simulink library "halout"  (R2021b)
settings: Solver=VariableStepAuto  StartTime=0.0  StopTime=10.0  RelTol=1e-3
undefined symbols (not defined in the file): C_TASK_5MS_S, FALSE, KHAL_CAN1FDAPS3E2E_flg, KHAL_CAN1FDAPS3TxReq_flg, KHAL_CAN1FDVCU2E2E_flg, KHAL_CAN1FDVCU2TxReq_flg, KHAL_CAN1FDVCU3E2E_flg, KHAL_CAN1FDVCU3TxReq_flg, KHAL_CAN1TxReq_flg, KHAL_CAN2TxReq_flg, KHAL_CAN3FDVCU1TxReq_flg, KHAL_CAN3FDVCU2E2E_flg, KHAL_CAN3FDVCU2TxReq_flg, KHAL_CAN3TxReq_flg, KHAL_CAN4FDVCU1E2E_flg, KHAL_CAN4FDVCU1TxReq_flg, KHAL_CAN4TxReq_flg, KHAL_CAN5TxReq_flg, ONE_INT, TRUE, ZERO_INT
libraries: FVT_lib x383, simulink x179
(part 11 of 20)

== system halout/HAL_OUT/CAN5/FD_VCU0_0x1F0 ==
  BSCP_outputs : Inport  OutDataTypeStr=Bus: BSCP_outputs
  BOUTP_outputs : Inport  Port=2  OutDataTypeStr=Bus: BOUTP_outputs
  EVCCAplusPwrUpReq : Subsystem
  FDADC12VDetAvg : Subsystem
  FrTqSource : Subsystem
  Ground{,1..8} (9 alike) : Ground
  HVRlyOpFail : Subsystem
  HVTHCMSysAvail : Subsystem
  LVBattChrgtimeAct : Subsystem
  LVBattVoltSta : Subsystem
  LVChrgHoldTAct : Subsystem
  LVSilentChrgLv : Subsystem
  LVSilentChrgReq : Subsystem
  LVSilentChrgSta : Subsystem
  MCUActDisFail : Subsystem
  PMMAllowECUSleep : Subsystem
  PowerDownFault : Subsystem
  PowerDownState : Subsystem
  PowerUpFault : Subsystem
  PowerUpState : Subsystem
  PwrDownReq : Subsystem
  PwrStaConstraint : Subsystem
  PwrStaONTOIVIPopReq : Subsystem
  PwrStaONTOIVIPopT : Subsystem
  PwrStaSelect : Subsystem
  PwrStaTOSta : Subsystem
  PwrUpReq : Subsystem
  RrTqSource : Subsystem
  SchedChgTOSta : Subsystem
  SilentChkAllowSleep : Subsystem
  SysAllowReadySta : Subsystem
  SysPwrSta : Subsystem
  TCountSta : Subsystem
  TimerAllowSleep : Subsystem
  VCUBrkSWSta : Subsystem
  VCUFLDoorSta : Subsystem
  VCUFRDoorSta : Subsystem
  VCURLDoorSta : Subsystem
  VCURRDoorSta : Subsystem
  VehHVPwrAvail4THCM : Subsystem
  bus_creator : BusCreator  Inputs=37  OutDataTypeStr=Bus: DT_CAN5_SG_FD_VCU0  NonVirtualBus=on
  bus_selector : BusSelector  OutputSignals=VOUTP_EvccAplusPwrUpReq_flg
  bus_selector1 : BusSelector  OutputSignals=VOUTP_FDADC12VDetAvg_mV
  bus_selector10 : BusSelector  OutputSignals=VOUTP_PMMAllowECUSleep_flg
  bus_selector11 : BusSelector  OutputSignals=VOUTP_PowerDownFault_enum
  bus_selector12 : BusSelector  OutputSignals=VOUTP_PowerDownState_enum
  bus_selector13 : BusSelector  OutputSignals=VOUTP_PowerUpFault_enum
  bus_selector14 : BusSelector  OutputSignals=VOUTP_PowerUpState_enum
  bus_selector15 : BusSelector  OutputSignals=VOUTP_PwrDownReq_enum
  bus_selector16 : BusSelector  OutputSignals=VOUTP_PwrStaConstraint_enum
  bus_selector17 : BusSelector  OutputSignals=VOUTP_PwrStaONTOPopReq_flg
  bus_selector18 : BusSelector  OutputSignals=VOUTP_IVIPwrStaONTOPopT_s
  bus_selector19 : BusSelector  OutputSignals=VOUTP_PwrStaSelect_enum
  bus_selector2 : BusSelector  OutputSignals=VOUTP_TqSourceFr_enum
  bus_selector20 : BusSelector  OutputSignals=VOUTP_PwrStaTOSta_enum
  bus_selector21 : BusSelector  OutputSignals=VOUTP_PwrUpReq_enum
  bus_selector22 : BusSelector  OutputSignals=VOUTP_TqSourceRr_enum
  bus_selector23 : BusSelector  OutputSignals=VOUTP_SilentChkAllowSleep_flg
  bus_selector24 : BusSelector  OutputSignals=VOUTP_SysPowerMode_enum
  bus_selector25 : BusSelector  OutputSignals=VOUTP_TCountSta_enum
  bus_selector26 : BusSelector  OutputSignals=VOUTP_TimerAllowSleep_flg
  bus_selector27 : BusSelector  OutputSignals=VOUTP_VehHVPwrAvail4THCM_W
  bus_selector3 : BusSelector  OutputSignals=VOUTP_HVTHCMSysAvail_enum
  bus_selector4 : BusSelector  OutputSignals=VOUTP_LVBattChrgTimeCnt_s
  bus_selector5 : BusSelector  OutputSignals=VOUTP_LVBattVoltSta_enum
  bus_selector6 : BusSelector  OutputSignals=VOUTP_LVChrgHoldTtimer_s
  bus_selector7 : BusSelector  OutputSignals=VOUTP_LVSilentChrgLv_enum
  bus_selector8 : BusSelector  OutputSignals=VOUTP_LVSilentChrgReq_flg
  bus_selector9 : BusSelector  OutputSignals=VOUTP_LVSilentChrgSta_enum
  FD_VCU0 : Outport
  wires:
  BSCP_outputs/1 -> [BSCP_outputs]
  BOUTP_outputs/1 -> [BOUTP_outputs]
  [CAN5_EVCCAplusPwrUpReq] -> bus_creator/1  "CAN5_EVCCAplusPwrUpReq"
  [CAN5_FDADC12VDetAvg] -> bus_creator/2  "CAN5_FDADC12VDetAvg"
  [CAN5_Fr_TqSource] -> bus_creator/3  "CAN5_Fr_TqSource"
  [CAN5_HVRlyOpFail] -> bus_creator/4  "CAN5_HVRlyOpFail"
  [CAN5_HVTHCMSysAvail] -> bus_creator/5  "CAN5_HVTHCMSysAvail"
  [CAN5_LVBattChrgtimeAct] -> bus_creator/6  "CAN5_LVBattChrgtimeAct"
  [CAN5_LVBattVoltSta] -> bus_creator/7  "CAN5_LVBattVoltSta"
  [CAN5_LVChrgHoldTAct] -> bus_creator/8  "CAN5_LVChrgHoldTAct"
  [CAN5_LVSilentChrgLv] -> bus_creator/9  "CAN5_LVSilentChrgLv"
  [CAN5_LVSilentChrgReq] -> bus_creator/10  "CAN5_LVSilentChrgReq"
  [CAN5_LVSilentChrgSta] -> bus_creator/11  "CAN5_LVSilentChrgSta"
  [CAN5_MCUActDisFail] -> bus_creator/12  "CAN5_MCUActDisFail"
  [CAN5_PMMAllowECUSleep] -> bus_creator/13  "CAN5_PMMAllowECUSleep"
  [CAN5_PowerDownFault] -> bus_creator/14  "CAN5_PowerDownFault"
  [CAN5_PowerDownState] -> bus_creator/15  "CAN5_PowerDownState"
  [CAN5_PowerUpFault] -> bus_creator/16  "CAN5_PowerUpFault"
  [CAN5_PowerUpState] -> bus_creator/17  "CAN5_PowerUpState"
  [CAN5_PwrDownReq] -> bus_creator/18  "CAN5_PwrDownReq"
  [CAN5_PwrStaConstraint] -> bus_creator/19  "CAN5_PwrStaConstraint"
  [CAN5_PwrStaONTOIVIPopReq] -> bus_creator/20  "CAN5_PwrStaONTOIVIPopReq"
  [CAN5_PwrStaONTOIVIPopT] -> bus_creator/21  "CAN5_PwrStaONTOIVIPopT"
  [CAN5_PwrStaSelect] -> bus_creator/22  "CAN5_PwrStaSelect"
  [CAN5_PwrStaTOSta] -> bus_creator/23  "CAN5_PwrStaTOSta"
  [CAN5_PwrUpReq] -> bus_creator/24  "CAN5_PwrUpReq"
  [CAN5_Rr_TqSource] -> bus_creator/25  "CAN5_Rr_TqSource"
  [CAN5_SchedChgTOSta] -> bus_creator/26  "CAN5_SchedChgTOSta"
  [CAN5_SilentChkAllowSleep] -> bus_creator/27  "CAN5_SilentChkAllowSleep"
  [CAN5_SysAllowReadySta] -> bus_creator/28  "CAN5_SysAllowReadySta"
  [CAN5_SysPwrSta] -> bus_creator/29  "CAN5_SysPwrSta"
  [CAN5_TCountSta] -> bus_creator/30  "CAN5_TCountSta"
  [CAN5_TimerAllowSleep] -> bus_creator/31  "CAN5_TimerAllowSleep"
  [CAN5_VCUBrkSWSta] -> bus_creator/32  "CAN5_VCUBrkSWSta"
  [CAN5_VCUFLDoorSta] -> bus_creator/33  "CAN5_VCUFLDoorSta"
  [CAN5_VCUFRDoorSta] -> bus_creator/34  "CAN5_VCUFRDoorSta"
  [CAN5_VCURLDoorSta] -> bus_creator/35  "CAN5_VCURLDoorSta"
  [CAN5_VCURRDoorSta] -> bus_creator/36  "CAN5_VCURRDoorSta"
  [CAN5_VehHVPwrAvail4THCM] -> bus_creator/37  "CAN5_VehHVPwrAvail4THCM"
  bus_creator/1 -> FD_VCU0/1
  EVCCAplusPwrUpReq/1(CAN5_EVCCAplusPwrUpReq) -> [CAN5_EVCCAplusPwrUpReq]
  FDADC12VDetAvg/1(CAN5_FDADC12VDetAvg) -> [CAN5_FDADC12VDetAvg]
  FrTqSource/1(CAN5_Fr_TqSource) -> [CAN5_Fr_TqSource]
  HVRlyOpFail/1(CAN5_HVRlyOpFail) -> [CAN5_HVRlyOpFail]
  HVTHCMSysAvail/1(CAN5_HVTHCMSysAvail) -> [CAN5_HVTHCMSysAvail]
  LVBattChrgtimeAct/1(CAN5_LVBattChrgtimeAct) -> [CAN5_LVBattChrgtimeAct]
  LVBattVoltSta/1(CAN5_LVBattVoltSta) -> [CAN5_LVBattVoltSta]
  LVChrgHoldTAct/1(CAN5_LVChrgHoldTAct) -> [CAN5_LVChrgHoldTAct]
  LVSilentChrgLv/1(CAN5_LVSilentChrgLv) -> [CAN5_LVSilentChrgLv]
  LVSilentChrgReq/1(CAN5_LVSilentChrgReq) -> [CAN5_LVSilentChrgReq]
  LVSilentChrgSta/1(CAN5_LVSilentChrgSta) -> [CAN5_LVSilentChrgSta]
  MCUActDisFail/1(CAN5_MCUActDisFail) -> [CAN5_MCUActDisFail]
  PMMAllowECUSleep/1(CAN5_PMMAllowECUSleep) -> [CAN5_PMMAllowECUSleep]
  PowerDownFault/1(CAN5_PowerDownFault) -> [CAN5_PowerDownFault]
  PowerDownState/1(CAN5_PowerDownState) -> [CAN5_PowerDownState]
  PowerUpFault/1(CAN5_PowerUpFault) -> [CAN5_PowerUpFault]
  PowerUpState/1(CAN5_PowerUpState) -> [CAN5_PowerUpState]
  PwrDownReq/1(CAN5_PwrDownReq) -> [CAN5_PwrDownReq]
  PwrStaConstraint/1(CAN5_PwrStaConstraint) -> [CAN5_PwrStaConstraint]
  PwrStaONTOIVIPopReq/1(CAN5_PwrStaONTOIVIPopReq) -> [CAN5_PwrStaONTOIVIPopReq]
  PwrStaONTOIVIPopT/1(CAN5_PwrStaONTOIVIPopT) -> [CAN5_PwrStaONTOIVIPopT]
  PwrStaSelect/1(CAN5_PwrStaSelect) -> [CAN5_PwrStaSelect]
  PwrStaTOSta/1(CAN5_PwrStaTOSta) -> [CAN5_PwrStaTOSta]
  PwrUpReq/1(CAN5_PwrUpReq) -> [CAN5_PwrUpReq]
  RrTqSource/1(CAN5_Rr_TqSource) -> [CAN5_Rr_TqSource]
  SchedChgTOSta/1(CAN5_SchedChgTOSta) -> [CAN5_SchedChgTOSta]
  SilentChkAllowSleep/1(CAN5_SilentChkAllowSleep) -> [CAN5_SilentChkAllowSleep]
  SysAllowReadySta/1(CAN5_SysAllowReadySta) -> [CAN5_SysAllowReadySta]
  SysPwrSta/1(CAN5_SysPwrSta) -> [CAN5_SysPwrSta]
  TCountSta/1(CAN5_TCountSta) -> [CAN5_TCountSta]
  TimerAllowSleep/1(CAN5_TimerAllowSleep) -> [CAN5_TimerAllowSleep]
  VCUBrkSWSta/1(CAN5_VCUBrkSWSta) -> [CAN5_VCUBrkSWSta]
  VCUFLDoorSta/1(CAN5_VCUFLDoorSta) -> [CAN5_VCUFLDoorSta]
  VCUFRDoorSta/1(CAN5_VCUFRDoorSta) -> [CAN5_VCUFRDoorSta]
  VCURLDoorSta/1(CAN5_VCURLDoorSta) -> [CAN5_VCURLDoorSta]
  VCURRDoorSta/1(CAN5_VCURRDoorSta) -> [CAN5_VCURRDoorSta]
  VehHVPwrAvail4THCM/1(CAN5_VehHVPwrAvail4THCM) -> [CAN5_VehHVPwrAvail4THCM]
  bus_selector/1 -> EVCCAplusPwrUpReq/1(EVCCAplusPwrUpReq)  "<VOUTP_EvccAplusPwrUpReq_flg>"
  [BOUTP_outputs] -> bus_selector/1
  bus_selector1/1 -> FDADC12VDetAvg/1(FDADC12VDetAvg)  "<VOUTP_FDADC12VDetAvg_mV>"
  [BOUTP_outputs] -> bus_selector1/1
  bus_selector2/1 -> FrTqSource/1(FrTqSource)  "<VOUTP_TqSourceFr_enum>"
  [BOUTP_outputs] -> bus_selector2/1
  Ground/1 -> HVRlyOpFail/1(HVRlyOpFail)
  bus_selector3/1 -> HVTHCMSysAvail/1(HVTHCMSysAvail)  "<VOUTP_HVTHCMSysAvail_enum>"
  [BOUTP_outputs] -> bus_selector3/1
  bus_selector4/1 -> LVBattChrgtimeAct/1(LVBattChrgtimeAct)  "<VOUTP_LVBattChrgTimeCnt_s>"
  [BOUTP_outputs] -> bus_selector4/1
  bus_selector5/1 -> LVBattVoltSta/1(LVBattVoltSta)  "<VOUTP_LVBattVoltSta_enum>"
  [BOUTP_outputs] -> bus_selector5/1
  bus_selector6/1 -> LVChrgHoldTAct/1(LVChrgHoldTAct)  "<VOUTP_LVChrgHoldTtimer_s>"
  [BOUTP_outputs] -> bus_selector6/1
  bus_selector7/1 -> LVSilentChrgLv/1(LVSilentChrgLv)  "<VOUTP_LVSilentChrgLv_enum>"
  [BOUTP_outputs] -> bus_selector7/1
  bus_selector8/1 -> LVSilentChrgReq/1(LVSilentChrgReq)  "<VOUTP_LVSilentChrgReq_flg>"
  [BOUTP_outputs] -> bus_selector8/1
  bus_selector9/1 -> LVSilentChrgSta/1(LVSilentChrgSta)  "<VOUTP_LVSilentChrgSta_enum>"
  [BOUTP_outputs] -> bus_selector9/1
  Ground1/1 -> MCUActDisFail/1(MCUActDisFail)
  bus_selector10/1 -> PMMAllowECUSleep/1(PMMAllowECUSleep)  "<VOUTP_PMMAllowECUSleep_flg>"
  [BOUTP_outputs] -> bus_selector10/1
  bus_selector11/1 -> PowerDownFault/1(PowerDownFault)  "<VOUTP_PowerDownFault_enum>"
  [BOUTP_outputs] -> bus_selector11/1
  bus_selector12/1 -> PowerDownState/1(PowerDownState)  "<VOUTP_PowerDownState_enum>"
  [BOUTP_outputs] -> bus_selector12/1
  bus_selector13/1 -> PowerUpFault/1(PowerUpFault)  "<VOUTP_PowerUpFault_enum>"
  [BOUTP_outputs] -> bus_selector13/1
  bus_selector14/1 -> PowerUpState/1(PowerUpState)  "<VOUTP_PowerUpState_enum>"
  [BOUTP_outputs] -> bus_selector14/1
  bus_selector15/1 -> PwrDownReq/1(PwrDownReq)  "<VOUTP_PwrDownReq_enum>"
  [BOUTP_outputs] -> bus_selector15/1
  bus_selector16/1 -> PwrStaConstraint/1(PwrStaConstraint)  "<VOUTP_PwrStaConstraint_enum>"
  [BOUTP_outputs] -> bus_selector16/1
  bus_selector17/1 -> PwrStaONTOIVIPopReq/1(PwrStaONTOIVIPopReq)  "<VOUTP_PwrStaONTOPopReq_flg>"
  [BOUTP_outputs] -> bus_selector17/1
  bus_selector18/1 -> PwrStaONTOIVIPopT/1(PwrStaONTOIVIPopT)  "<VOUTP_IVIPwrStaONTOPopT_s>"
  [BOUTP_outputs] -> bus_selector18/1
  bus_selector19/1 -> PwrStaSelect/1(PwrStaSelect)  "<VOUTP_PwrStaSelect_enum>"
  [BOUTP_outputs] -> bus_selector19/1
  bus_selector20/1 -> PwrStaTOSta/1(PwrStaTOSta)  "<VOUTP_PwrStaTOSta_enum>"
  [BOUTP_outputs] -> bus_selector20/1
  bus_selector21/1 -> PwrUpReq/1(PwrUpReq)  "<VOUTP_PwrUpReq_enum>"
  [BOUTP_outputs] -> bus_selector21/1
  bus_selector22/1 -> RrTqSource/1(RrTqSource)  "<VOUTP_TqSourceRr_enum>"
  [BOUTP_outputs] -> bus_selector22/1
  Ground2/1 -> SchedChgTOSta/1(SchedChgTOSta)
  bus_selector23/1 -> SilentChkAllowSleep/1(SilentChkAllowSleep)  "<VOUTP_SilentChkAllowSleep_flg>"
  [BOUTP_outputs] -> bus_selector23/1
  Ground3/1 -> SysAllowReadySta/1(SysAllowReadySta)
  bus_selector24/1 -> SysPwrSta/1(SysPwrSta)  "<VOUTP_SysPowerMode_enum>"
  [BOUTP_outputs] -> bus_selector24/1
  bus_selector25/1 -> TCountSta/1(TCountSta)  "<VOUTP_TCountSta_enum>"
  [BOUTP_outputs] -> bus_selector25/1
  bus_selector26/1 -> TimerAllowSleep/1(TimerAllowSleep)  "<VOUTP_TimerAllowSleep_flg>"
  [BOUTP_outputs] -> bus_selector26/1
  Ground4/1 -> VCUBrkSWSta/1(VCUBrkSWSta)
  Ground5/1 -> VCUFLDoorSta/1(VCUFLDoorSta)
  Ground6/1 -> VCUFRDoorSta/1(VCUFRDoorSta)
  Ground7/1 -> VCURLDoorSta/1(VCURLDoorSta)
  Ground8/1 -> VCURRDoorSta/1(VCURRDoorSta)
  bus_selector27/1 -> VehHVPwrAvail4THCM/1(VehHVPwrAvail4THCM)  "<VOUTP_VehHVPwrAvail4THCM_W>"
  [BOUTP_outputs] -> bus_selector27/1

== system halout/HAL_OUT/CAN5/FD_VCU1_0x116 ==
  BSCP_outputs : Inport  OutDataTypeStr=Bus: BSCP_outputs
  BOUTP_outputs : Inport  Port=2  OutDataTypeStr=Bus: BOUTP_outputs
  MSACrlSta : Subsystem
  PwrSta : Subsystem
  ShiftGearPosn : Subsystem
  bus_creator : BusCreator  Inputs=3  OutDataTypeStr=Bus: DT_CAN5_SG_FD_VCU1  NonVirtualBus=on
  bus_selector : BusSelector  OutputSignals=VOUTP_MSACtrlSta_enum
  bus_selector1 : BusSelector  OutputSignals=VOUTP_PowerSta_enum
  bus_selector2 : BusSelector  OutputSignals=VOUTP_ShiftGearPosn_enum
  FD_VCU1 : Outport
  wires:
  BSCP_outputs/1 -> [BSCP_outputs]
  BOUTP_outputs/1 -> [BOUTP_outputs]
  [CAN5_MSA_Crl_Sta] -> bus_creator/1  "CAN5_MSA_Crl_Sta"
  [CAN5_PwrSta] -> bus_creator/2  "CAN5_PwrSta"
  [CAN5_ShiftGearPosn] -> bus_creator/3  "CAN5_ShiftGearPosn"
  bus_creator/1 -> FD_VCU1/1
  MSACrlSta/1(CAN5_MSA_Crl_Sta) -> [CAN5_MSA_Crl_Sta]
  PwrSta/1(CAN5_PwrSta) -> [CAN5_PwrSta]
  ShiftGearPosn/1(CAN5_ShiftGearPosn) -> [CAN5_ShiftGearPosn]
  bus_selector/1 -> MSACrlSta/1(MSACrlSta)  "<VOUTP_MSACtrlSta_enum>"
  [BOUTP_outputs] -> bus_selector/1
  bus_selector1/1 -> PwrSta/1(PwrSta)  "<VOUTP_PowerSta_enum>"
  [BOUTP_outputs] -> bus_selector1/1
  bus_selector2/1 -> ShiftGearPosn/1(ShiftGearPosn)  "<VOUTP_ShiftGearPosn_enum>"
  [BOUTP_outputs] -> bus_selector2/1

== system halout/HAL_OUT/CAN5/FD_VCU3_0x159 ==
  BSCP_outputs : Inport  OutDataTypeStr=Bus: BSCP_outputs
  BOUTP_outputs : Inport  Port=2  OutDataTypeStr=Bus: BOUTP_outputs
  CSVCU3CAN1 : Subsystem
  EquivAccPedalSWSta : Subsystem
  FrEDUActTqValid : Subsystem
  FrEDUAvailBrkRgnTq : Subsystem
  FrEDUAvailBrkRgnTqValid : Subsystem
  FrEDURealARgnTq : Subsystem
  FrEDURealDrvOrBRgnTq : Subsystem
  FrEDURolRgnTqValid : Subsystem
  FrEDUSpd : Subsystem
  FrEDUSpdValid : Subsystem
  FrRgnDecrSta : Subsystem
  FrRgnPermSta : Subsystem
  Ground{,1..5} (6 alike) : Ground
  PTCSPermSta : Subsystem
  RCVCU3CAN1 : Subsystem
  RgnAbnorSta : Subsystem
  RrEDUActTqValid : Subsystem
  RrEDUAvailBrkRgnTq : Subsystem
  RrEDUAvailBrkRgnTqValid : Subsystem
  RrEDURealARgnTq : Subsystem
  RrEDURealDrvOrBRgnTq : Subsystem
  RrEDURolRgnTqValid : Subsystem
  RrEDUSpd : Subsystem
  RrEDUSpdValid : Subsystem
  RrRgnDecrSta : Subsystem
  RrRgnPermSta : Subsystem
  bus_creator : BusCreator  Inputs=25  OutDataTypeStr=Bus: DT_CAN5_SG_FD_VCU3  NonVirtualBus=on
  bus_selector : BusSelector  OutputSignals=VOUTP_EquivAccPedalSWSta_flg
  bus_selector1 : BusSelector  OutputSignals=VOUTP_FrEDUAvailBrkRgnTq_Nm
  bus_selector10 : BusSelector  OutputSignals=VOUTP_RgnAbnorSta_flg
  bus_selector11 : BusSelector  OutputSignals=VOUTP_RrEDUAvailBrkRgnTq_Nm
  bus_selector12 : BusSelector  OutputSignals=VOUTP_RrEDUAvailBrkRgnTqV_flg
  bus_selector13 : BusSelector  OutputSignals=VOUTP_RrEDURolRgnTq_Nm
  bus_selector14 : BusSelector  OutputSignals=VOUTP_RrEDUActTq_Nm
  bus_selector15 : BusSelector  OutputSignals=VOUTP_RrEDUSpd_rpm
  bus_selector16 : BusSelector  OutputSignals=VOUTP_RrEDUSpdValid_flg
  bus_selector17 : BusSelector  OutputSignals=VOUTP_RrRgnDecrSta_flg
  bus_selector18 : BusSelector  OutputSignals=VOUTP_RrRgnPermSta_flg
  bus_selector2 : BusSelector  OutputSignals=VOUTP_FrEDUAvailBrkRgnTqV_flg
  bus_selector3 : BusSelector  OutputSignals=VOUTP_FrEDURolRgnTq_Nm
  bus_selector4 : BusSelector  OutputSignals=VOUTP_FrEDUActTq_Nm
  bus_selector5 : BusSelector  OutputSignals=VOUTP_FrEDUSpd_rpm
  bus_selector6 : BusSelector  OutputSignals=VOUTP_FrEDUSpdValid_flg
  bus_selector7 : BusSelector  OutputSignals=VOUTP_FrRgnDecrSta_flg
  bus_selector8 : BusSelector  OutputSignals=VOUTP_FrRgnPermSta_flg
  bus_selector9 : BusSelector  OutputSignals=VOUTP_PTCSPermSta_flg
  FD_VCU3 : Outport
  wires:
  BSCP_outputs/1 -> [BSCP_outputs]
  BOUTP_outputs/1 -> [BOUTP_outputs]
  [CAN5_CS_VCU3_CAN1] -> bus_creator/1  "CAN5_CS_VCU3_CAN1"
  [CAN5_EquivAccPedalSWSta] -> bus_creator/2  "CAN5_EquivAccPedalSWSta"
  [CAN5_Fr_EDUActTqValid] -> bus_creator/3  "CAN5_Fr_EDUActTqValid"
  [CAN5_Fr_EDUAvailBrkRgnTq] -> bus_creator/4  "CAN5_Fr_EDUAvailBrkRgnTq"
  [CAN5_Fr_EDUAvailBrkRgnTqValid] -> bus_creator/5  "CAN5_Fr_EDUAvailBrkRgnTqValid"
  [CAN5_Fr_EDURealARgnTq] -> bus_creator/6  "CAN5_Fr_EDURealARgnTq"
  [CAN5_Fr_EDURealDrvOrBRgnTq] -> bus_creator/7  "CAN5_Fr_EDURealDrvOrBRgnTq"
  [CAN5_Fr_EDURolRgnTqValid] -> bus_creator/8  "CAN5_Fr_EDURolRgnTqValid"
  [CAN5_Fr_EDUSpd] -> bus_creator/9  "CAN5_Fr_EDUSpd"
  [CAN5_Fr_EDUSpdValid] -> bus_creator/10  "CAN5_Fr_EDUSpdValid"
  [CAN5_Fr_RgnDecrSta] -> bus_creator/11  "CAN5_Fr_RgnDecrSta"
  [CAN5_Fr_RgnPermSta] -> bus_creator/12  "CAN5_Fr_RgnPermSta"
  [CAN5_PTCS_PermSta] -> bus_creator/13  "CAN5_PTCS_PermSta"
  [CAN5_RC_VCU3_CAN1] -> bus_creator/14  "CAN5_RC_VCU3_CAN1"
  [CAN5_RgnAbnorSta] -> bus_creator/15  "CAN5_RgnAbnorSta"
  [CAN5_Rr_EDUActTqValid] -> bus_creator/16  "CAN5_Rr_EDUActTqValid"
  [CAN5_Rr_EDUAvailBrkRgnTq] -> bus_creator/17  "CAN5_Rr_EDUAvailBrkRgnTq"
  [CAN5_Rr_EDUAvailBrkRgnTqValid] -> bus_creator/18  "CAN5_Rr_EDUAvailBrkRgnTqValid"
  [CAN5_Rr_EDURealARgnTq] -> bus_creator/19  "CAN5_Rr_EDURealARgnTq"
  [CAN5_Rr_EDURealDrvOrBRgnTq] -> bus_creator/20  "CAN5_Rr_EDURealDrvOrBRgnTq"
  [CAN5_Rr_EDURolRgnTqValid] -> bus_creator/21  "CAN5_Rr_EDURolRgnTqValid"
  [CAN5_Rr_EDUSpd] -> bus_creator/22  "CAN5_Rr_EDUSpd"
  [CAN5_Rr_EDUSpdValid] -> bus_creator/23  "CAN5_Rr_EDUSpdValid"
  [CAN5_Rr_RgnDecrSta] -> bus_creator/24  "CAN5_Rr_RgnDecrSta"
  [CAN5_Rr_RgnPermSta] -> bus_creator/25  "CAN5_Rr_RgnPermSta"
  bus_creator/1 -> FD_VCU3/1
  CSVCU3CAN1/1(CAN5_CS_VCU3_CAN1) -> [CAN5_CS_VCU3_CAN1]
  EquivAccPedalSWSta/1(CAN5_EquivAccPedalSWSta) -> [CAN5_EquivAccPedalSWSta]
  FrEDUActTqValid/1(CAN5_Fr_EDUActTqValid) -> [CAN5_Fr_EDUActTqValid]
  FrEDUAvailBrkRgnTq/1(CAN5_Fr_EDUAvailBrkRgnTq) -> [CAN5_Fr_EDUAvailBrkRgnTq]
  FrEDUAvailBrkRgnTqValid/1(CAN5_Fr_EDUAvailBrkRgnTqValid) -> [CAN5_Fr_EDUAvailBrkRgnTqValid]
  FrEDURealARgnTq/1(CAN5_Fr_EDURealARgnTq) -> [CAN5_Fr_EDURealARgnTq]
  FrEDURealDrvOrBRgnTq/1(CAN5_Fr_EDURealDrvOrBRgnTq) -> [CAN5_Fr_EDURealDrvOrBRgnTq]
  FrEDURolRgnTqValid/1(CAN5_Fr_EDURolRgnTqValid) -> [CAN5_Fr_EDURolRgnTqValid]
  FrEDUSpd/1(CAN5_Fr_EDUSpd) -> [CAN5_Fr_EDUSpd]
  FrEDUSpdValid/1(CAN5_Fr_EDUSpdValid) -> [CAN5_Fr_EDUSpdValid]
  FrRgnDecrSta/1(CAN5_Fr_RgnDecrSta) -> [CAN5_Fr_RgnDecrSta]
  FrRgnPermSta/1(CAN5_Fr_RgnPermSta) -> [CAN5_Fr_RgnPermSta]
  PTCSPermSta/1(CAN5_PTCS_PermSta) -> [CAN5_PTCS_PermSta]
  RCVCU3CAN1/1(CAN5_RC_VCU3_CAN1) -> [CAN5_RC_VCU3_CAN1]
  RgnAbnorSta/1(CAN5_RgnAbnorSta) -> [CAN5_RgnAbnorSta]
  RrEDUActTqValid/1(CAN5_Rr_EDUActTqValid) -> [CAN5_Rr_EDUActTqValid]
  RrEDUAvailBrkRgnTq/1(CAN5_Rr_EDUAvailBrkRgnTq) -> [CAN5_Rr_EDUAvailBrkRgnTq]
  RrEDUAvailBrkRgnTqValid/1(CAN5_Rr_EDUAvailBrkRgnTqValid) -> [CAN5_Rr_EDUAvailBrkRgnTqValid]
  RrEDURealARgnTq/1(CAN5_Rr_EDURealARgnTq) -> [CAN5_Rr_EDURealARgnTq]
  RrEDURealDrvOrBRgnTq/1(CAN5_Rr_EDURealDrvOrBRgnTq) -> [CAN5_Rr_EDURealDrvOrBRgnTq]
  RrEDURolRgnTqValid/1(CAN5_Rr_EDURolRgnTqValid) -> [CAN5_Rr_EDURolRgnTqValid]
  RrEDUSpd/1(CAN5_Rr_EDUSpd) -> [CAN5_Rr_EDUSpd]
  RrEDUSpdValid/1(CAN5_Rr_EDUSpdValid) -> [CAN5_Rr_EDUSpdValid]
  RrRgnDecrSta/1(CAN5_Rr_RgnDecrSta) -> [CAN5_Rr_RgnDecrSta]
  RrRgnPermSta/1(CAN5_Rr_RgnPermSta) -> [CAN5_Rr_RgnPermSta]
  Ground/1 -> CSVCU3CAN1/1(CSVCU3CAN1)
  bus_selector/1 -> EquivAccPedalSWSta/1(EquivAccPedalSWSta)  "<VOUTP_EquivAccPedalSWSta_flg>"
  [BOUTP_outputs] -> bus_selector/1
  Ground1/1 -> FrEDUActTqValid/1(FrEDUActTqValid)
  bus_selector1/1 -> FrEDUAvailBrkRgnTq/1(FrEDUAvailBrkRgnTq)  "<VOUTP_FrEDUAvailBrkRgnTq_Nm>"
  [BOUTP_outputs] -> bus_selector1/1
  bus_selector2/1 -> FrEDUAvailBrkRgnTqValid/1(FrEDUAvailBrkRgnTqValid)  "<VOUTP_FrEDUAvailBrkRgnTqV_flg>"
  [BOUTP_outputs] -> bus_selector2/1
  bus_selector3/1 -> FrEDURealARgnTq/1(FrEDURealARgnTq)  "<VOUTP_FrEDURolRgnTq_Nm>"
  [BOUTP_outputs] -> bus_selector3/1
  bus_selector4/1 -> FrEDURealDrvOrBRgnTq/1(FrEDURealDrvOrBRgnTq)  "<VOUTP_FrEDUActTq_Nm>"
  [BOUTP_outputs] -> bus_selector4/1
  Ground2/1 -> FrEDURolRgnTqValid/1(FrEDURolRgnTqValid)
  bus_selector5/1 -> FrEDUSpd/1(FrEDUSpd)  "<VOUTP_FrEDUSpd_rpm>"
  [BOUTP_outputs] -> bus_selector5/1
  bus_selector6/1 -> FrEDUSpdValid/1(FrEDUSpdValid)  "<VOUTP_FrEDUSpdValid_flg>"
  [BOUTP_outputs] -> bus_selector6/1
  bus_selector7/1 -> FrRgnDecrSta/1(FrRgnDecrSta)  "<VOUTP_FrRgnDecrSta_flg>"
  [BOUTP_outputs] -> bus_selector7/1
  bus_selector8/1 -> FrRgnPermSta/1(FrRgnPermSta)  "<VOUTP_FrRgnPermSta_flg>"
  [BOUTP_outputs] -> bus_selector8/1
  bus_selector9/1 -> PTCSPermSta/1(PTCSPermSta)  "<VOUTP_PTCSPermSta_flg>"
  [BOUTP_outputs] -> bus_selector9/1
  Ground3/1 -> RCVCU3CAN1/1(RCVCU3CAN1)
  bus_selector10/1 -> RgnAbnorSta/1(RgnAbnorSta)  "<VOUTP_RgnAbnorSta_flg>"
  [BOUTP_outputs] -> bus_selector10/1
  Ground4/1 -> RrEDUActTqValid/1(RrEDUActTqValid)
  bus_selector11/1 -> RrEDUAvailBrkRgnTq/1(RrEDUAvailBrkRgnTq)  "<VOUTP_RrEDUAvailBrkRgnTq_Nm>"
  [BOUTP_outputs] -> bus_selector11/1
  bus_selector12/1 -> RrEDUAvailBrkRgnTqValid/1(RrEDUAvailBrkRgnTqValid)  "<VOUTP_RrEDUAvailBrkRgnTqV_flg>"
  [BOUTP_outputs] -> bus_selector12/1
  bus_selector13/1 -> RrEDURealARgnTq/1(RrEDURealARgnTq)  "<VOUTP_RrEDURolRgnTq_Nm>"
  [BOUTP_outputs] -> bus_selector13/1
  bus_selector14/1 -> RrEDURealDrvOrBRgnTq/1(RrEDURealDrvOrBRgnTq)  "<VOUTP_RrEDUActTq_Nm>"
  [BOUTP_outputs] -> bus_selector14/1
  Ground5/1 -> RrEDURolRgnTqValid/1(RrEDURolRgnTqValid)
  bus_selector15/1 -> RrEDUSpd/1(RrEDUSpd)  "<VOUTP_RrEDUSpd_rpm>"
  [BOUTP_outputs] -> bus_selector15/1
  bus_selector16/1 -> RrEDUSpdValid/1(RrEDUSpdValid)  "<VOUTP_RrEDUSpdValid_flg>"
  [BOUTP_outputs] -> bus_selector16/1
  bus_selector17/1 -> RrRgnDecrSta/1(RrRgnDecrSta)  "<VOUTP_RrRgnDecrSta_flg>"
  [BOUTP_outputs] -> bus_selector17/1
  bus_selector18/1 -> RrRgnPermSta/1(RrRgnPermSta)  "<VOUTP_RrRgnPermSta_flg>"
  [BOUTP_outputs] -> bus_selector18/1

== system halout/HAL_OUT/CAN5/FD_VCU4_0x3C0 ==
  BSCP_outputs : Inport  OutDataTypeStr=Bus: BSCP_outputs
  BOUTP_outputs : Inport  Port=2  OutDataTypeStr=Bus: BOUTP_outputs
  EngAGSCloseSta : Subsystem
  EngActvDmpDisabSta : Subsystem
  EngCoastDwSta : Subsystem
  EngPwrLockSta : Subsystem
  Ground : Ground
  Ground1 : Ground
  Ground2 : Ground
  VehMalfunLevel : Subsystem
  bus_creator : BusCreator  Inputs=5  OutDataTypeStr=Bus: DT_CAN5_SG_FD_VCU4  NonVirtualBus=on
  bus_selector : BusSelector  OutputSignals=VOUTP_IVIPwrLockSta_enum
  bus_selector1 : BusSelector  OutputSignals=VOUTP_VehMalfunLevel_enum
  FD_VCU4 : Outport
  wires:
  BSCP_outputs/1 -> [BSCP_outputs]
  BOUTP_outputs/1 -> [BOUTP_outputs]
  [CAN5_Eng_AGSCloseSta] -> bus_creator/1  "CAN5_Eng_AGSCloseSta"
  [CAN5_Eng_ActvDmpDisabSta] -> bus_creator/2  "CAN5_Eng_ActvDmpDisabSta"
  [CAN5_Eng_CoastDwSta] -> bus_creator/3  "CAN5_Eng_CoastDwSta"
  [CAN5_Eng_PwrLockSta] -> bus_creator/4  "CAN5_Eng_PwrLockSta"
  [CAN5_VehMalfunLevel] -> bus_creator/5  "CAN5_VehMalfunLevel"
  bus_creator/1 -> FD_VCU4/1
  EngAGSCloseSta/1(CAN5_Eng_AGSCloseSta) -> [CAN5_Eng_AGSCloseSta]
  EngActvDmpDisabSta/1(CAN5_Eng_ActvDmpDisabSta) -> [CAN5_Eng_ActvDmpDisabSta]
  EngCoastDwSta/1(CAN5_Eng_CoastDwSta) -> [CAN5_Eng_CoastDwSta]
  EngPwrLockSta/1(CAN5_Eng_PwrLockSta) -> [CAN5_Eng_PwrLockSta]
  VehMalfunLevel/1(CAN5_VehMalfunLevel) -> [CAN5_VehMalfunLevel]
  Ground/1 -> EngAGSCloseSta/1(EngAGSCloseSta)
  Ground1/1 -> EngActvDmpDisabSta/1(EngActvDmpDisabSta)
  Ground2/1 -> EngCoastDwSta/1(EngCoastDwSta)
  bus_selector/1 -> EngPwrLockSta/1(EngPwrLockSta)  "<VOUTP_IVIPwrLockSta_enum>"
  [BOUTP_outputs] -> bus_selector/1
  bus_selector1/1 -> VehMalfunLevel/1(VehMalfunLevel)  "<VOUTP_VehMalfunLevel_enum>"
  [BOUTP_outputs] -> bus_selector1/1

== system halout/HAL_OUT/CAN5/FD_VCU5_0x245 ==
  BSCP_outputs : Inport  OutDataTypeStr=Bus: BSCP_outputs
  BOUTP_outputs : Inport  Port=2  OutDataTypeStr=Bus: BOUTP_outputs
  EDriveSysErrAccPedalErr : Subsystem
  EDriveSysErrMCUErr : Subsystem
  EDriveSysErrShifterErr : Subsystem
  EDriveSysErrVCUErr : Subsystem
  Ground{,1..6} (7 alike) : Ground
  HVSysErrIsolationErr : Subsystem
  HVSysErrPackErr : Subsystem
  HVSysErrRelayErr : Subsystem
  LVSysErrPwrOutpErr : Subsystem
  LimphomeAct : Subsystem
  LowSOCWarn : Subsystem
  PwrStaErr : Subsystem
  ReVehThdChkSta : Subsystem
  bus_creator : BusCreator  Inputs=12  OutDataTypeStr=Bus: DT_CAN5_SG_FD_VCU5  NonVirtualBus=on
  bus_selector : BusSelector  OutputSignals=VOUTP_EDriveSysErr_VCUErrTmp_flg
  bus_selector1 : BusSelector  OutputSignals=VOUTP_LVSysErrPwrOutErr_flg
  bus_selector2 : BusSelector  OutputSignals=VOUTP_LimpHomeActTmp_flg
  bus_selector3 : BusSelector  OutputSignals=VOUTP_LowSOCWarn_enum
  bus_selector4 : BusSelector  OutputSignals=VOUTP_ReVehThdChkSta_enum
  FD_VCU5 : Outport
  wires:
  BSCP_outputs/1 -> [BSCP_outputs]
  BOUTP_outputs/1 -> [BOUTP_outputs]
  [CAN5_EDriveSysErr_AccPedalErr] -> bus_creator/1  "CAN5_EDriveSysErr_AccPedalErr"
  [CAN5_EDriveSysErr_MCUErr] -> bus_creator/2  "CAN5_EDriveSysErr_MCUErr"
  [CAN5_EDriveSysErr_ShifterErr] -> bus_creator/3  "CAN5_EDriveSysErr_ShifterErr"
  [CAN5_EDriveSysErr_VCUErr] -> bus_creator/4  "CAN5_EDriveSysErr_VCUErr"
  [CAN5_HVSysErr_IsolationErr] -> bus_creator/5  "CAN5_HVSysErr_IsolationErr"
  [CAN5_HVSysErr_PackErr] -> bus_creator/6  "CAN5_HVSysErr_PackErr"
  [CAN5_HVSysErr_RelayErr] -> bus_creator/7  "CAN5_HVSysErr_RelayErr"
  [CAN5_LVSysErr_PwrOutpErr] -> bus_creator/8  "CAN5_LVSysErr_PwrOutpErr"
  [CAN5_LimphomeAct] -> bus_creator/9  "CAN5_LimphomeAct"
  [CAN5_LowSOCWarn] -> bus_creator/10  "CAN5_LowSOCWarn"
  [CAN5_PwrStaErr] -> bus_creator/11  "CAN5_PwrStaErr"
  [CAN5_Re_VehThdChkSta] -> bus_creator/12  "CAN5_Re_VehThdChkSta"
  bus_creator/1 -> FD_VCU5/1
  EDriveSysErrAccPedalErr/1(CAN5_EDriveSysErr_AccPedalErr) -> [CAN5_EDriveSysErr_AccPedalErr]
  EDriveSysErrMCUErr/1(CAN5_EDriveSysErr_MCUErr) -> [CAN5_EDriveSysErr_MCUErr]
  EDriveSysErrShifterErr/1(CAN5_EDriveSysErr_ShifterErr) -> [CAN5_EDriveSysErr_ShifterErr]
  EDriveSysErrVCUErr/1(CAN5_EDriveSysErr_VCUErr) -> [CAN5_EDriveSysErr_VCUErr]
  HVSysErrIsolationErr/1(CAN5_HVSysErr_IsolationErr) -> [CAN5_HVSysErr_IsolationErr]
  HVSysErrPackErr/1(CAN5_HVSysErr_PackErr) -> [CAN5_HVSysErr_PackErr]
  HVSysErrRelayErr/1(CAN5_HVSysErr_RelayErr) -> [CAN5_HVSysErr_RelayErr]
  LVSysErrPwrOutpErr/1(CAN5_LVSysErr_PwrOutpErr) -> [CAN5_LVSysErr_PwrOutpErr]
  LimphomeAct/1(CAN5_LimphomeAct) -> [CAN5_LimphomeAct]
  LowSOCWarn/1(CAN5_LowSOCWarn) -> [CAN5_LowSOCWarn]
  PwrStaErr/1(CAN5_PwrStaErr) -> [CAN5_PwrStaErr]
  ReVehThdChkSta/1(CAN5_Re_VehThdChkSta) -> [CAN5_Re_VehThdChkSta]
  Ground/1 -> EDriveSysErrAccPedalErr/1(EDriveSysErrAccPedalErr)
  Ground1/1 -> EDriveSysErrMCUErr/1(EDriveSysErrMCUErr)
  Ground2/1 -> EDriveSysErrShifterErr/1(EDriveSysErrShifterErr)
  bus_selector/1 -> EDriveSysErrVCUErr/1(EDriveSysErrVCUErr)  "<VOUTP_EDriveSysErr_VCUErrTmp_flg>"
  [BOUTP_outputs] -> bus_selector/1
  Ground3/1 -> HVSysErrIsolationErr/1(HVSysErrIsolationErr)
  Ground4/1 -> HVSysErrPackErr/1(HVSysErrPackErr)
  Ground5/1 -> HVSysErrRelayErr/1(HVSysErrRelayErr)
  bus_selector1/1 -> LVSysErrPwrOutpErr/1(LVSysErrPwrOutpErr)  "<VOUTP_LVSysErrPwrOutErr_flg>"
  [BOUTP_outputs] -> bus_selector1/1
  bus_selector2/1 -> LimphomeAct/1(LimphomeAct)  "<VOUTP_LimpHomeActTmp_flg>"
  [BOUTP_outputs] -> bus_selector2/1
  bus_selector3/1 -> LowSOCWarn/1(LowSOCWarn)  "<VOUTP_LowSOCWarn_enum>"
  [BOUTP_outputs] -> bus_selector3/1
  Ground6/1 -> PwrStaErr/1(PwrStaErr)
  bus_selector4/1 -> ReVehThdChkSta/1(ReVehThdChkSta)  "<VOUTP_ReVehThdChkSta_enum>"
  [BOUTP_outputs] -> bus_selector4/1

== system halout/HAL_OUT/CAN1/FD_APS1_0x236/APSAngleTarget ==
  APSAngleTarget : Inport
  Data Type Conversion : DataTypeConversion  OutDataTypeStr=uint16  RndMeth=Round
  convert_out : FVT_lib/hal/convert_out  gain=0.1  offset=-900
  CAN1_APS_Angle_Target : Outport
  wires:
  Data Type Conversion/1 -> CAN1_APS_Angle_Target/1
  convert_out/1 -> Data Type Conversion/1
  APSAngleTarget/1 -> convert_out/1

== system halout/HAL_OUT/CAN1/FD_APS1_0x236/APSRqEPASCtrl ==
  APSRqEPASCtrl : Inport
  Data Type Conversion : DataTypeConversion  OutDataTypeStr=uint8  RndMeth=Round
  CAN1_APS_Rq_EPAS_Ctrl : Outport
  wires:
  Data Type Conversion/1 -> CAN1_APS_Rq_EPAS_Ctrl/1
  APSRqEPASCtrl/1 -> Data Type Conversion/1

== system halout/HAL_OUT/CAN1/FD_APS1_0x236/APSStaSystem ==
  APSStaSystem : Inport
  Data Type Conversion : DataTypeConversion  OutDataTypeStr=uint8  RndMeth=Round
  CAN1_APS_Sta_System : Outport
  wires:
  Data Type Conversion/1 -> CAN1_APS_Sta_System/1
  APSStaSystem/1 -> Data Type Conversion/1

== system halout/HAL_OUT/CAN1/FD_APS1_0x236/APSVRqEPASCtrl ==
  APSVRqEPASCtrl : Inport
  Data Type Conversion : DataTypeConversion  OutDataTypeStr=uint8  RndMeth=Round
  CAN1_APS_V_Rq_EPAS_Ctrl : Outport
  wires:
  Data Type Conversion/1 -> CAN1_APS_V_Rq_EPAS_Ctrl/1
  APSVRqEPASCtrl/1 -> Data Type Conversion/1

== system halout/HAL_OUT/CAN1/FD_APS2_0x210/APSDFLL ==
  APSDFLL : Inport
  Data Type Conversion : DataTypeConversion  OutDataTypeStr=uint16  RndMeth=Round
  CAN1_APS_D_FLL : Outport
  wires:
  Data Type Conversion/1 -> CAN1_APS_D_FLL/1
  APSDFLL/1 -> Data Type Conversion/1

== system halout/HAL_OUT/CAN1/FD_APS2_0x210/APSDFLR ==
  APSDFLR : Inport
  Data Type Conversion : DataTypeConversion  OutDataTypeStr=uint16  RndMeth=Round
  CAN1_APS_D_FLR : Outport
  wires:
  Data Type Conversion/1 -> CAN1_APS_D_FLR/1
  APSDFLR/1 -> Data Type Conversion/1

== system halout/HAL_OUT/CAN1/FD_APS2_0x210/APSDRLL ==
  APSDRLL : Inport
  Data Type Conversion : DataTypeConversion  OutDataTypeStr=uint16  RndMeth=Round
  CAN1_APS_D_RLL : Outport
  wires:
  Data Type Conversion/1 -> CAN1_APS_D_RLL/1
  APSDRLL/1 -> Data Type Conversion/1

== system halout/HAL_OUT/CAN1/FD_APS2_0x210/APSDRLR ==
  APSDRLR : Inport
  Data Type Conversion : DataTypeConversion  OutDataTypeStr=uint16  RndMeth=Round
  CAN1_APS_D_RLR : Outport
  wires:
  Data Type Conversion/1 -> CAN1_APS_D_RLR/1
  APSDRLR/1 -> Data Type Conversion/1

== system halout/HAL_OUT/CAN1/FD_APS2_0x210/APSExitCondition ==
  APSExitCondition : Inport
  Data Type Conversion : DataTypeConversion  OutDataTypeStr=uint8  RndMeth=Round
  CAN1_APS_ExitCondition : Outport
  wires:
  Data Type Conversion/1 -> CAN1_APS_ExitCondition/1
  APSExitCondition/1 -> Data Type Conversion/1

== system halout/HAL_OUT/CAN1/FD_APS2_0x210/APSHWVer ==
  APSHWVer : Inport
  Data Type Conversion : DataTypeConversion  OutDataTypeStr=uint8  RndMeth=Round
  CAN1_APS_HW_Ver : Outport
  wires:
  Data Type Conversion/1 -> CAN1_APS_HW_Ver/1
  APSHWVer/1 -> Data Type Conversion/1

== system halout/HAL_OUT/CAN1/FD_APS2_0x210/APSProgressPCT ==
  APSProgressPCT : Inport
  Data Type Conversion : DataTypeConversion  OutDataTypeStr=uint8  RndMeth=Round
  CAN1_APS_Progress_PCT : Outport
  wires:
  Data Type Conversion/1 -> CAN1_APS_Progress_PCT/1
  APSProgressPCT/1 -> Data Type Conversion/1

== system halout/HAL_OUT/CAN1/FD_APS2_0x210/APSRQDisplay ==
  APSRQDisplay : Inport
  Data Type Conversion : DataTypeConversion  OutDataTypeStr=uint8  RndMeth=Round
  CAN1_APS_RQ_Display : Outport
  wires:
  Data Type Conversion/1 -> CAN1_APS_RQ_Display/1
  APSRQDisplay/1 -> Data Type Conversion/1

== system halout/HAL_OUT/CAN1/FD_APS2_0x210/APSSWVer ==
  APSSWVer : Inport
  Data Type Conversion : DataTypeConversion  OutDataTypeStr=uint8  RndMeth=Round
  CAN1_APS_SW_Ver : Outport
  wires:
  Data Type Conversion/1 -> CAN1_APS_SW_Ver/1
  APSSWVer/1 -> Data Type Conversion/1

== system halout/HAL_OUT/CAN1/FD_APS2_0x210/PASAFCL ==
  PASAFCL : Inport
  Data Type Conversion : DataTypeConversion  OutDataTypeStr=uint8  RndMeth=Round
  CAN1_PAS_A_FCL : Outport
  wires:
  Data Type Conversion/1 -> CAN1_PAS_A_FCL/1
  PASAFCL/1 -> Data Type Conversion/1

== system halout/HAL_OUT/CAN1/FD_APS2_0x210/PASAFCR ==
  PASAFCR : Inport
  Data Type Conversion : DataTypeConversion  OutDataTypeStr=uint8  RndMeth=Round
  CAN1_PAS_A_FCR : Outport
  wires:
  Data Type Conversion/1 -> CAN1_PAS_A_FCR/1
  PASAFCR/1 -> Data Type Conversion/1

== system halout/HAL_OUT/CAN1/FD_APS2_0x210/PASAFML ==
  PASAFML : Inport
  Data Type Conversion : DataTypeConversion  OutDataTypeStr=uint8  RndMeth=Round
  CAN1_PAS_A_FML : Outport
  wires:
  Data Type Conversion/1 -> CAN1_PAS_A_FML/1
  PASAFML/1 -> Data Type Conversion/1

== system halout/HAL_OUT/CAN1/FD_APS2_0x210/PASAFMR ==
  PASAFMR : Inport
  Data Type Conversion : DataTypeConversion  OutDataTypeStr=uint8  RndMeth=Round
  CAN1_PAS_A_FMR : Outport
  wires:
  Data Type Conversion/1 -> CAN1_PAS_A_FMR/1
  PASAFMR/1 -> Data Type Conversion/1

== system halout/HAL_OUT/CAN1/FD_APS2_0x210/PASARCL ==
  PASARCL : Inport
  Data Type Conversion : DataTypeConversion  OutDataTypeStr=uint8  RndMeth=Round
  CAN1_PAS_A_RCL : Outport
  wires:
  Data Type Conversion/1 -> CAN1_PAS_A_RCL/1
  PASARCL/1 -> Data Type Conversion/1

== system halout/HAL_OUT/CAN1/FD_APS2_0x210/PASARCR ==
  PASARCR : Inport
  Data Type Conversion : DataTypeConversion  OutDataTypeStr=uint8  RndMeth=Round
  CAN1_PAS_A_RCR : Outport
  wires:
  Data Type Conversion/1 -> CAN1_PAS_A_RCR/1
  PASARCR/1 -> Data Type Conversion/1

== system halout/HAL_OUT/CAN1/FD_APS2_0x210/PASARML ==
  PASARML : Inport
  Data Type Conversion : DataTypeConversion  OutDataTypeStr=uint8  RndMeth=Round
  CAN1_PAS_A_RML : Outport
  wires:
  Data Type Conversion/1 -> CAN1_PAS_A_RML/1
  PASARML/1 -> Data Type Conversion/1

== system halout/HAL_OUT/CAN1/FD_APS2_0x210/PASARMR ==
  PASARMR : Inport
  Data Type Conversion : DataTypeConversion  OutDataTypeStr=uint8  RndMeth=Round
  CAN1_PAS_A_RMR : Outport
  wires:
  Data Type Conversion/1 -> CAN1_PAS_A_RMR/1
  PASARMR/1 -> Data Type Conversion/1

== system halout/HAL_OUT/CAN1/FD_APS2_0x210/PASChime ==
  PASChime : Inport
  Data Type Conversion : DataTypeConversion  OutDataTypeStr=uint8  RndMeth=Round
  CAN1_PAS_Chime : Outport
  wires:
  Data Type Conversion/1 -> CAN1_PAS_Chime/1
  PASChime/1 -> Data Type Conversion/1

== system halout/HAL_OUT/CAN1/FD_APS2_0x210/PASDFCL ==
  PASDFCL : Inport
  Data Type Conversion : DataTypeConversion  OutDataTypeStr=uint8  RndMeth=Round
  CAN1_PAS_D_FCL : Outport
  wires:
  Data Type Conversion/1 -> CAN1_PAS_D_FCL/1
  PASDFCL/1 -> Data Type Conversion/1

== system halout/HAL_OUT/CAN1/FD_APS2_0x210/PASDFCR ==
  PASDFCR : Inport
  Data Type Conversion : DataTypeConversion  OutDataTypeStr=uint8  RndMeth=Round
  CAN1_PAS_D_FCR : Outport
  wires:
  Data Type Conversion/1 -> CAN1_PAS_D_FCR/1
  PASDFCR/1 -> Data Type Conversion/1

== system halout/HAL_OUT/CAN1/FD_APS2_0x210/PASDFML ==
  PASDFML : Inport
  Data Type Conversion : DataTypeConversion  OutDataTypeStr=uint8  RndMeth=Round
  CAN1_PAS_D_FML : Outport
  wires:
  Data Type Conversion/1 -> CAN1_PAS_D_FML/1
  PASDFML/1 -> Data Type Conversion/1

== system halout/HAL_OUT/CAN1/FD_APS2_0x210/PASDFMR ==
  PASDFMR : Inport
  Data Type Conversion : DataTypeConversion  OutDataTypeStr=uint8  RndMeth=Round
  CAN1_PAS_D_FMR : Outport
  wires:
  Data Type Conversion/1 -> CAN1_PAS_D_FMR/1
  PASDFMR/1 -> Data Type Conversion/1

== system halout/HAL_OUT/CAN1/FD_APS2_0x210/PASDRCL ==
  PASDRCL : Inport
  Data Type Conversion : DataTypeConversion  OutDataTypeStr=uint8  RndMeth=Round
  CAN1_PAS_D_RCL : Outport
  wires:
  Data Type Conversion/1 -> CAN1_PAS_D_RCL/1
  PASDRCL/1 -> Data Type Conversion/1

== system halout/HAL_OUT/CAN1/FD_APS2_0x210/PASDRCR ==
  PASDRCR : Inport
  Data Type Conversion : DataTypeConversion  OutDataTypeStr=uint8  RndMeth=Round
  CAN1_PAS_D_RCR : Outport
  wires:
  Data Type Conversion/1 -> CAN1_PAS_D_RCR/1
  PASDRCR/1 -> Data Type Conversion/1

== system halout/HAL_OUT/CAN1/FD_APS2_0x210/PASDRML ==
  PASDRML : Inport
  Data Type Conversion : DataTypeConversion  OutDataTypeStr=uint8  RndMeth=Round
  CAN1_PAS_D_RML : Outport
  wires:
  Data Type Conversion/1 -> CAN1_PAS_D_RML/1
  PASDRML/1 -> Data Type Conversion/1

== system halout/HAL_OUT/CAN1/FD_APS2_0x210/PASDRMR ==
  PASDRMR : Inport
  Data Type Conversion : DataTypeConversion  OutDataTypeStr=uint8  RndMeth=Round
  CAN1_PAS_D_RMR : Outport
  wires:
  Data Type Conversion/1 -> CAN1_PAS_D_RMR/1
  PASDRMR/1 -> Data Type Conversion/1

== system halout/HAL_OUT/CAN1/FD_APS2_0x210/PASModOperation ==
  PASModOperation : Inport
  Data Type Conversion : DataTypeConversion  OutDataTypeStr=uint8  RndMeth=Round
  CAN1_PAS_Mod_Operation : Outport
  wires:
  Data Type Conversion/1 -> CAN1_PAS_Mod_Operation/1
  PASModOperation/1 -> Data Type Conversion/1

== system halout/HAL_OUT/CAN1/FD_APS2_0x210/PASSNSRLayout ==
  PASSNSRLayout : Inport
  Data Type Conversion : DataTypeConversion  OutDataTypeStr=uint8  RndMeth=Round
  CAN1_PAS_SNSR_Layout : Outport
  wires:
  Data Type Conversion/1 -> CAN1_PAS_SNSR_Layout/1
  PASSNSRLayout/1 -> Data Type Conversion/1

== system halout/HAL_OUT/CAN1/FD_APS2_0x210/PASStaFSys ==
  PASStaFSys : Inport
  Data Type Conversion : DataTypeConversion  OutDataTypeStr=uint8  RndMeth=Round
  CAN1_PAS_Sta_F_Sys : Outport
  wires:
  Data Type Conversion/1 -> CAN1_PAS_Sta_F_Sys/1
  PASStaFSys/1 -> Data Type Conversion/1

== system halout/HAL_OUT/CAN1/FD_APS2_0x210/USSStaFCL ==
  USSStaFCL : Inport
  Data Type Conversion : DataTypeConversion  OutDataTypeStr=uint8  RndMeth=Round
  CAN1_USS_Sta_FCL : Outport
  wires:
  Data Type Conversion/1 -> CAN1_USS_Sta_FCL/1
  USSStaFCL/1 -> Data Type Conversion/1

== system halout/HAL_OUT/CAN1/FD_APS2_0x210/USSStaFCR ==
  USSStaFCR : Inport
  Data Type Conversion : DataTypeConversion  OutDataTypeStr=uint8  RndMeth=Round
  CAN1_USS_Sta_FCR : Outport
  wires:
  Data Type Conversion/1 -> CAN1_USS_Sta_FCR/1
  USSStaFCR/1 -> Data Type Conversion/1

== system halout/HAL_OUT/CAN1/FD_APS2_0x210/USSStaFLL ==
  USSStaFLL : Inport
  Data Type Conversion : DataTypeConversion  OutDataTypeStr=uint8  RndMeth=Round
  CAN1_USS_Sta_FLL : Outport
  wires:
  Data Type Conversion/1 -> CAN1_USS_Sta_FLL/1
  USSStaFLL/1 -> Data Type Conversion/1

== system halout/HAL_OUT/CAN1/FD_APS2_0x210/USSStaFLR ==
  USSStaFLR : Inport
  Data Type Conversion : DataTypeConversion  OutDataTypeStr=uint8  RndMeth=Round
  CAN1_USS_Sta_FLR : Outport
  wires:
  Data Type Conversion/1 -> CAN1_USS_Sta_FLR/1
  USSStaFLR/1 -> Data Type Conversion/1

== system halout/HAL_OUT/CAN1/FD_APS2_0x210/USSStaFML ==
  USSStaFML : Inport
  Data Type Conversion : DataTypeConversion  OutDataTypeStr=uint8  RndMeth=Round
  CAN1_USS_Sta_FML : Outport
  wires:
  Data Type Conversion/1 -> CAN1_USS_Sta_FML/1
  USSStaFML/1 -> Data Type Conversion/1

== system halout/HAL_OUT/CAN1/FD_APS2_0x210/USSStaFMR ==
  USSStaFMR : Inport
  Data Type Conversion : DataTypeConversion  OutDataTypeStr=uint8  RndMeth=Round
  CAN1_USS_Sta_FMR : Outport
  wires:
  Data Type Conversion/1 -> CAN1_USS_Sta_FMR/1
  USSStaFMR/1 -> Data Type Conversion/1

== system halout/HAL_OUT/CAN1/FD_APS2_0x210/USSStaRCL ==
  USSStaRCL : Inport
  Data Type Conversion : DataTypeConversion  OutDataTypeStr=uint8  RndMeth=Round
  CAN1_USS_Sta_RCL : Outport
  wires:
  Data Type Conversion/1 -> CAN1_USS_Sta_RCL/1
  USSStaRCL/1 -> Data Type Conversion/1

== system halout/HAL_OUT/CAN1/FD_APS2_0x210/USSStaRCR ==
  USSStaRCR : Inport
  Data Type Conversion : DataTypeConversion  OutDataTypeStr=uint8  RndMeth=Round
  CAN1_USS_Sta_RCR : Outport
  wires:
  Data Type Conversion/1 -> CAN1_USS_Sta_RCR/1
  USSStaRCR/1 -> Data Type Conversion/1

== system halout/HAL_OUT/CAN1/FD_APS2_0x210/USSStaRLL ==
  USSStaRLL : Inport
  Data Type Conversion : DataTypeConversion  OutDataTypeStr=uint8  RndMeth=Round
  CAN1_USS_Sta_RLL : Outport
  wires:
  Data Type Conversion/1 -> CAN1_USS_Sta_RLL/1
  USSStaRLL/1 -> Data Type Conversion/1

== system halout/HAL_OUT/CAN1/FD_APS2_0x210/USSStaRLR ==
  USSStaRLR : Inport
  Data Type Conversion : DataTypeConversion  OutDataTypeStr=uint8  RndMeth=Round
  CAN1_USS_Sta_RLR : Outport
  wires:
  Data Type Conversion/1 -> CAN1_USS_Sta_RLR/1
  USSStaRLR/1 -> Data Type Conversion/1

== system halout/HAL_OUT/CAN1/FD_APS2_0x210/USSStaRML ==
  USSStaRML : Inport
  Data Type Conversion : DataTypeConversion  OutDataTypeStr=uint8  RndMeth=Round
  CAN1_USS_Sta_RML : Outport
  wires:
  Data Type Conversion/1 -> CAN1_USS_Sta_RML/1
  USSStaRML/1 -> Data Type Conversion/1

== system halout/HAL_OUT/CAN1/FD_APS2_0x210/USSStaRMR ==
  USSStaRMR : Inport
  Data Type Conversion : DataTypeConversion  OutDataTypeStr=uint8  RndMeth=Round
  CAN1_USS_Sta_RMR : Outport
  wires:
  Data Type Conversion/1 -> CAN1_USS_Sta_RMR/1
  USSStaRMR/1 -> Data Type Conversion/1

== system halout/HAL_OUT/CAN1/FD_APS3_0x238/APS3LifeCount ==
  APS3LifeCount : Inport
  Data Type Conversion : DataTypeConversion  OutDataTypeStr=uint8  RndMeth=Round
  CAN1_APS3_LifeCount : Outport
  wires:
  Data Type Conversion/1 -> CAN1_APS3_LifeCount/1
  APS3LifeCount/1 -> Data Type Conversion/1

== system halout/HAL_OUT/CAN1/FD_APS3_0x238/APS3checksum ==
  APS3checksum : Inport
  Data Type Conversion : DataTypeConversion  OutDataTypeStr=uint8  RndMeth=Round
  CAN1_APS3_checksum : Outport
  wires:
  Data Type Conversion/1 -> CAN1_APS3_checksum/1
  APS3checksum/1 -> Data Type Conversion/1

== system halout/HAL_OUT/CAN1/FD_APS3_0x238/APSDecReq ==
  APSDecReq : Inport
  Data Type Conversion : DataTypeConversion  OutDataTypeStr=uint8  RndMeth=Round
  convert_out : FVT_lib/hal/convert_out  gain=0.1  offset=0
  CAN1_APS_DecReq : Outport
  wires:
  Data Type Conversion/1 -> CAN1_APS_DecReq/1
  convert_out/1 -> Data Type Conversion/1
  APSDecReq/1 -> convert_out/1

== system halout/HAL_OUT/CAN1/FD_APS3_0x238/APSDecReqA ==
  APSDecReqA : Inport
  Data Type Conversion : DataTypeConversion  OutDataTypeStr=uint8  RndMeth=Round
  CAN1_APS_DecReq_A : Outport
  wires:
  Data Type Conversion/1 -> CAN1_APS_DecReq_A/1
  APSDecReqA/1 -> Data Type Conversion/1

== system halout/HAL_OUT/CAN1/FD_APS3_0x238/APSOpenPTG ==
  APSOpenPTG : Inport
  Data Type Conversion : DataTypeConversion  OutDataTypeStr=uint8  RndMeth=Round
  CAN1_APSOpenPTG : Outport
  wires:
  Data Type Conversion/1 -> CAN1_APSOpenPTG/1
  APSOpenPTG/1 -> Data Type Conversion/1

== system halout/HAL_OUT/CAN1/FD_APS3_0x238/APSReq ==
  APSReq : Inport
  Data Type Conversion : DataTypeConversion  OutDataTypeStr=uint8  RndMeth=Round
  CAN1_APS_Req : Outport
  wires:
  Data Type Conversion/1 -> CAN1_APS_Req/1
  APSReq/1 -> Data Type Conversion/1

== system halout/HAL_OUT/CAN1/FD_APS3_0x238/Byte_0 ==
  APSOpenPTG : Inport
  APS_DecReq_A : Inport  Port=2
  CAAS_Sta : Inport  Port=3
  SPTGDet : Inport  Port=4
  BitwiseOR : simulink/Logic and Bit Operations/Bitwise Operator  logicop=OR  UseBitMask=off  NumInputPorts=4  BitMask=bin2dec('11011001')  BitMaskRealWorld=Stored Integer
  SignalPack : FVT_lib/hal/SignalPack  RightShiftCnt=0  BitMask=2^1-1  LeftShiftCnt=5
  SignalPack1 : FVT_lib/hal/SignalPack  RightShiftCnt=0  BitMask=2^1-1  LeftShiftCnt=3
  SignalPack2 : FVT_lib/hal/SignalPack  RightShiftCnt=0  BitMask=2^3-1  LeftShiftCnt=0
  SignalPack3 : FVT_lib/hal/SignalPack  RightShiftCnt=0  BitMask=2^1-1  LeftShiftCnt=4
  UnitConverter{,1..7} (8 alike) : DataTypeConversion  OutDataTypeStr=uint8  RndMeth=Round
  Byte_0 : Outport
  wires:
  BitwiseOR/1 -> Byte_0/1
  UnitConverter/1 -> BitwiseOR/1
  SignalPack/1 -> UnitConverter/1
  UnitConverter1/1 -> SignalPack/1
  APSOpenPTG/1 -> UnitConverter1/1
  UnitConverter2/1 -> BitwiseOR/2
  SignalPack1/1 -> UnitConverter2/1
  UnitConverter3/1 -> SignalPack1/1
  APS_DecReq_A/1 -> UnitConverter3/1
  UnitConverter4/1 -> BitwiseOR/3
  SignalPack2/1 -> UnitConverter4/1
  UnitConverter5/1 -> SignalPack2/1
  CAAS_Sta/1 -> UnitConverter5/1
  UnitConverter6/1 -> BitwiseOR/4
  SignalPack3/1 -> UnitConverter6/1
  UnitConverter7/1 -> SignalPack3/1
  SPTGDet/1 -> UnitConverter7/1

== system halout/HAL_OUT/CAN1/FD_APS3_0x238/Byte_1 ==
  APS_DecReq : Inport
  BitwiseOR : simulink/Logic and Bit Operations/Bitwise Operator  logicop=OR  UseBitMask=off  BitMask=bin2dec('11011001')  BitMaskRealWorld=Stored Integer
  SignalPack : FVT_lib/hal/SignalPack  RightShiftCnt=0  BitMask=2^8-1  LeftShiftCnt=0
  UnitConverter : DataTypeConversion  OutDataTypeStr=uint8  RndMeth=Round
  UnitConverter1 : DataTypeConversion  OutDataTypeStr=uint8  RndMeth=Round
  convert_out : FVT_lib/hal/convert_out  gain=0.1  offset=0
  Byte_1 : Outport
  wires:
  BitwiseOR/1 -> Byte_1/1
  UnitConverter/1 -> BitwiseOR/1
  SignalPack/1 -> UnitConverter/1
  UnitConverter1/1 -> SignalPack/1
  convert_out/1 -> UnitConverter1/1
  APS_DecReq/1 -> convert_out/1

== system halout/HAL_OUT/CAN1/FD_APS3_0x238/Byte_2 ==
  APS_Req : Inport
  SPTG_Sta : Inport  Port=2
  BitwiseOR : simulink/Logic and Bit Operations/Bitwise Operator  logicop=OR  UseBitMask=off  NumInputPorts=2  BitMask=bin2dec('11011001')  BitMaskRealWorld=Stored Integer
  SignalPack : FVT_lib/hal/SignalPack  RightShiftCnt=0  BitMask=2^3-1  LeftShiftCnt=0
  SignalPack1 : FVT_lib/hal/SignalPack  RightShiftCnt=0  BitMask=2^3-1  LeftShiftCnt=3
  UnitConverter{,1..3} (4 alike) : DataTypeConversion  OutDataTypeStr=uint8  RndMeth=Round
  Byte_2 : Outport
  wires:
  BitwiseOR/1 -> Byte_2/1
  UnitConverter/1 -> BitwiseOR/1
  SignalPack/1 -> UnitConverter/1
  UnitConverter1/1 -> SignalPack/1
  APS_Req/1 -> UnitConverter1/1
  UnitConverter2/1 -> BitwiseOR/2
  SignalPack1/1 -> UnitConverter2/1
  UnitConverter3/1 -> SignalPack1/1
  SPTG_Sta/1 -> UnitConverter3/1

== system halout/HAL_OUT/CAN1/FD_APS3_0x238/Byte_6 ==
  APS3_LifeCount : Inport
  BitwiseOR : simulink/Logic and Bit Operations/Bitwise Operator  logicop=OR  UseBitMask=off  BitMask=bin2dec('11011001')  BitMaskRealWorld=Stored Integer
  SignalPack : FVT_lib/hal/SignalPack  RightShiftCnt=0  BitMask=2^4-1  LeftShiftCnt=4
  UnitConverter : DataTypeConversion  OutDataTypeStr=uint8  RndMeth=Round
  UnitConverter1 : DataTypeConversion  OutDataTypeStr=uint8  RndMeth=Round
  Byte_6 : Outport
  wires:
  BitwiseOR/1 -> Byte_6/1
  UnitConverter/1 -> BitwiseOR/1
  SignalPack/1 -> UnitConverter/1
  UnitConverter1/1 -> SignalPack/1
  APS3_LifeCount/1 -> UnitConverter1/1

== system halout/HAL_OUT/CAN1/FD_APS3_0x238/Byte_7 ==
  APS3_checksum : Inport
  BitwiseOR : simulink/Logic and Bit Operations/Bitwise Operator  logicop=OR  UseBitMask=off  BitMask=bin2dec('11011001')  BitMaskRealWorld=Stored Integer
  SignalPack : FVT_lib/hal/SignalPack  RightShiftCnt=0  BitMask=2^8-1  LeftShiftCnt=0
  UnitConverter : DataTypeConversion  OutDataTypeStr=uint8  RndMeth=Round
  UnitConverter1 : DataTypeConversion  OutDataTypeStr=uint8  RndMeth=Round
  Byte_7 : Outport
  wires:
  BitwiseOR/1 -> Byte_7/1
  UnitConverter/1 -> BitwiseOR/1
  SignalPack/1 -> UnitConverter/1
  UnitConverter1/1 -> SignalPack/1
  APS3_checksum/1 -> UnitConverter1/1

== system halout/HAL_OUT/CAN1/FD_APS3_0x238/CAASSta ==
  CAASSta : Inport
  Data Type Conversion : DataTypeConversion  OutDataTypeStr=uint8  RndMeth=Round
  CAN1_CAAS_Sta : Outport
  wires:
  Data Type Conversion/1 -> CAN1_CAAS_Sta/1
  CAASSta/1 -> Data Type Conversion/1

== system halout/HAL_OUT/CAN1/FD_APS3_0x238/SPTGDet ==
  SPTGDet : Inport
  Data Type Conversion : DataTypeConversion  OutDataTypeStr=uint8  RndMeth=Round
  CAN1_SPTGDet : Outport
  wires:
  Data Type Conversion/1 -> CAN1_SPTGDet/1
  SPTGDet/1 -> Data Type Conversion/1

== system halout/HAL_OUT/CAN1/FD_APS3_0x238/SPTGSta ==
  SPTGSta : Inport
  Data Type Conversion : DataTypeConversion  OutDataTypeStr=uint8  RndMeth=Round
  CAN1_SPTG_Sta : Outport
  wires:
  Data Type Conversion/1 -> CAN1_SPTG_Sta/1
  SPTGSta/1 -> Data Type Conversion/1

== system halout/HAL_OUT/CAN1/FD_BCM1_0x216/AllDoorSW ==
  AllDoorSW : Inport
  Data Type Conversion : DataTypeConversion  OutDataTypeStr=uint8  RndMeth=Round
  CAN1_AllDoorSW : Outport
  wires:
  Data Type Conversion/1 -> CAN1_AllDoorSW/1
  AllDoorSW/1 -> Data Type Conversion/1

== system halout/HAL_OUT/CAN1/FD_BCM1_0x216/AntiTheftSeatFold ==
  AntiTheftSeatFold : Inport
  Data Type Conversion : DataTypeConversion  OutDataTypeStr=uint8  RndMeth=Round
  CAN1_AntiTheftSeatFold : Outport
  wires:
  Data Type Conversion/1 -> CAN1_AntiTheftSeatFold/1
  AntiTheftSeatFold/1 -> Data Type Conversion/1

== system halout/HAL_OUT/CAN1/FD_BCM1_0x216/AntitheftSta ==
  AntitheftSta : Inport
  Data Type Conversion : DataTypeConversion  OutDataTypeStr=uint8  RndMeth=Round
  CAN1_AntitheftSta : Outport
  wires:
  Data Type Conversion/1 -> CAN1_AntitheftSta/1
  AntitheftSta/1 -> Data Type Conversion/1

== system halout/HAL_OUT/CAN1/FD_BCM1_0x216/BCMBuzzerReq ==
  BCMBuzzerReq : Inport
  Data Type Conversion : DataTypeConversion  OutDataTypeStr=uint8  RndMeth=Round
  CAN1_BCM_Buzzer_Req : Outport
  wires:
  Data Type Conversion/1 -> CAN1_BCM_Buzzer_Req/1
  BCMBuzzerReq/1 -> Data Type Conversion/1

== system halout/HAL_OUT/CAN1/FD_BCM1_0x216/BCMDoorLockSta ==
  BCMDoorLockSta : Inport
  Data Type Conversion : DataTypeConversion  OutDataTypeStr=uint8  RndMeth=Round
  CAN1_BCM_DoorLock_Sta : Outport
  wires:
  Data Type Conversion/1 -> CAN1_BCM_DoorLock_Sta/1
  BCMDoorLockSta/1 -> Data Type Conversion/1

== system halout/HAL_OUT/CAN1/FD_BCM1_0x216/BrakeLamp ==
  BrakeLamp : Inport
  Data Type Conversion : DataTypeConversion  OutDataTypeStr=uint8  RndMeth=Round
  CAN1_BrakeLamp : Outport
  wires:
  Data Type Conversion/1 -> CAN1_BrakeLamp/1
  BrakeLamp/1 -> Data Type Conversion/1
